simulink model "task_02_simulink"  (R2024b)
settings: Solver=VariableStepAuto  StartTime=0.0  StopTime=10.0  RelTol=1e-3
settings Model: Creator=jx2004  LastModifiedBy=jx2004

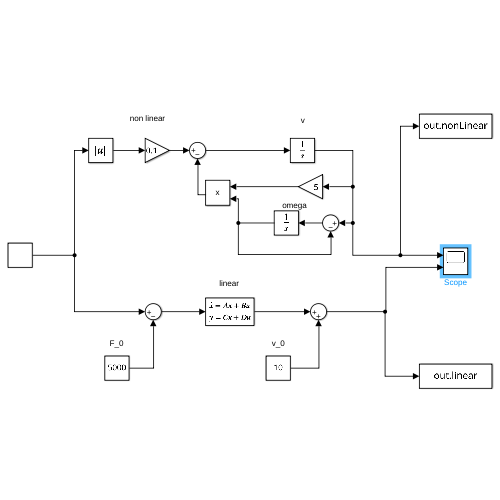
[thumbnail: Simulink's stored preview of the top-level diagram]
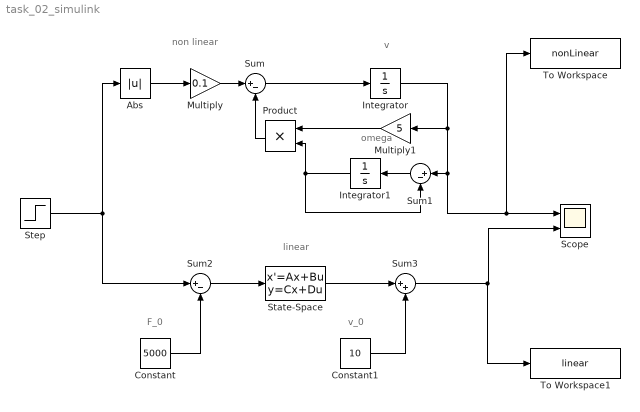
== system task_02_simulink ==
  note: v_0
  note: F_0
  note: linear
  note: omega
  note: v
  note: non linear
  Abs : Abs  SaturateOnIntegerOverflow=off
  Constant : Constant  Value=5000
  Constant1 : Constant  Value=10
  Integrator : Integrator  InitialCondition=10
  Integrator1 : Integrator  InitialCondition=10
  Multiply : Gain  Gain=0.1
  Multiply1 : Gain  Gain=5
  Product : Product
  Scope : Scope  NumInputPorts=2
  State-Space : StateSpace  A=[-50 -50; 1 -1]  B=[0.1; 0]  C=[1 0]  D=0  InitialCondition=0
  Step : Step  Before=5000  After=5010  SampleTime=0
  Sum : Sum  Inputs=|+-
  Sum1 : Sum  Inputs=|+-
  Sum2 : Sum  Inputs=|+-
  Sum3 : Sum  Inputs=|++
  To Workspace : ToWorkspace  VariableName=nonLinear  SaveFormat=Timeseries  SampleTime=-1
  To Workspace1 : ToWorkspace  VariableName=linear  SaveFormat=Timeseries  SampleTime=-1
  wires:
  Step/1 -> Abs/1, Sum2/1
  Abs/1 -> Multiply/1
  Integrator/1 -> Sum1/1, To Workspace/1, Scope/1, Multiply1/1
  Multiply1/1 -> Product/1
  Sum1/1 -> Integrator1/1
  Integrator1/1 -> Product/2, Sum1/2
  Sum2/1 -> State-Space/1
  State-Space/1 -> Sum3/1
  Sum3/1 -> To Workspace1/1, Scope/2
  Constant1/1 -> Sum3/2
  Constant/1 -> Sum2/2
  Multiply/1 -> Sum/1
  Sum/1 -> Integrator/1
  Product/1 -> Sum/2
